simulink model "ECE371_Lab6"  (R2017a)
settings: Solver=ode3  StartTime=0.0  StopTime=Tf  FixedStep=0.01  RelTol=1e-3
settings Model: Creator=localmgr  LastModifiedBy=localmgr

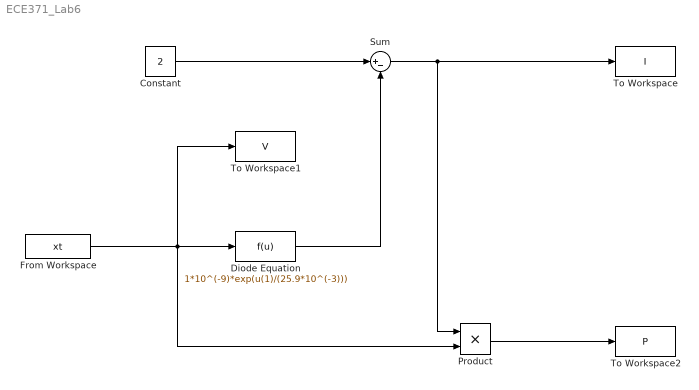
== system ECE371_Lab6 ==
  Constant : Constant  Value=2
  "Diode Equation " : Fcn  Expr=1*10^(-9)*exp(u(1)/(25.9*10^(-3)))
  From Workspace : FromWorkspace  VariableName=xt  SampleTime=0
  Product : Product
  Sum : Sum  Inputs=|+-
  To Workspace : ToWorkspace  VariableName=I  SaveFormat=Timeseries  SampleTime=-1
  To Workspace1 : ToWorkspace  VariableName=V  SaveFormat=Timeseries  SampleTime=-1
  To Workspace2 : ToWorkspace  VariableName=P  SaveFormat=Timeseries  SampleTime=-1
  wires:
  Constant/1 -> Sum/1
  Sum/1 -> To Workspace/1, Product/1
  From Workspace/1 -> To Workspace1/1, "Diode Equation "/1, Product/2
  "Diode Equation "/1 -> Sum/2
  Product/1 -> To Workspace2/1
